simulink model "shift_register_100"  (R2018b)
settings: Solver=FixedStepAuto  StartTime=0.0  StopTime=500*(15e-9)  FixedStep=15e-9  RelTol=1e-3
settings Model: Creator=meyer  LastModifiedBy=jason
settings OptimizationCC: DefaultParameterBehavior=Inlined

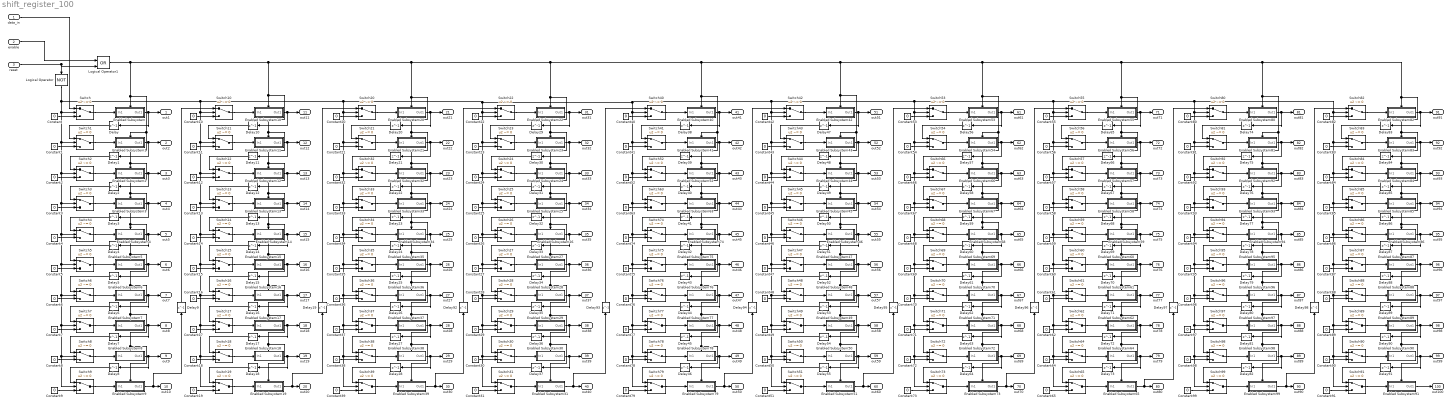
== system shift_register_100 ==
  data_in : Inport  OutDataTypeStr=fixdt(1,16,15)
  enable : Inport  Port=2
  reset : Inport  Port=3
  Constant{,1..99} (100 alike) : Constant  Value=0  OutDataTypeStr=Inherit: Inherit via back propagation  SampleTime=-1
  Delay{,1..98} (99 alike) : Delay  DelayLength=1
  Enabled Subsystem : Subsystem  TreatAsAtomicUnit=on
  Enabled Subsystem1 : Subsystem  TreatAsAtomicUnit=on
  Enabled Subsystem10 : Subsystem  TreatAsAtomicUnit=on
  Enabled Subsystem11 : Subsystem  TreatAsAtomicUnit=on
  Enabled Subsystem12 : Subsystem  TreatAsAtomicUnit=on
  Enabled Subsystem13 : Subsystem  TreatAsAtomicUnit=on
  Enabled Subsystem14 : Subsystem  TreatAsAtomicUnit=on
  Enabled Subsystem15 : Subsystem  TreatAsAtomicUnit=on
  Enabled Subsystem16 : Subsystem  TreatAsAtomicUnit=on
  Enabled Subsystem17 : Subsystem  TreatAsAtomicUnit=on
  Enabled Subsystem18 : Subsystem  TreatAsAtomicUnit=on
  Enabled Subsystem19 : Subsystem  TreatAsAtomicUnit=on
  Enabled Subsystem2 : Subsystem  TreatAsAtomicUnit=on
  Enabled Subsystem20 : Subsystem  TreatAsAtomicUnit=on
  Enabled Subsystem21 : Subsystem  TreatAsAtomicUnit=on
  Enabled Subsystem22 : Subsystem  TreatAsAtomicUnit=on
  Enabled Subsystem23 : Subsystem  TreatAsAtomicUnit=on
  Enabled Subsystem24 : Subsystem  TreatAsAtomicUnit=on
  Enabled Subsystem25 : Subsystem  TreatAsAtomicUnit=on
  Enabled Subsystem26 : Subsystem  TreatAsAtomicUnit=on
  Enabled Subsystem27 : Subsystem  TreatAsAtomicUnit=on
  Enabled Subsystem28 : Subsystem  TreatAsAtomicUnit=on
  Enabled Subsystem29 : Subsystem  TreatAsAtomicUnit=on
  Enabled Subsystem3 : Subsystem  TreatAsAtomicUnit=on
  Enabled Subsystem30 : Subsystem  TreatAsAtomicUnit=on
  Enabled Subsystem31 : Subsystem  TreatAsAtomicUnit=on
  Enabled Subsystem32 : Subsystem  TreatAsAtomicUnit=on
  Enabled Subsystem33 : Subsystem  TreatAsAtomicUnit=on
  Enabled Subsystem34 : Subsystem  TreatAsAtomicUnit=on
  Enabled Subsystem35 : Subsystem  TreatAsAtomicUnit=on
  Enabled Subsystem36 : Subsystem  TreatAsAtomicUnit=on
  Enabled Subsystem37 : Subsystem  TreatAsAtomicUnit=on
  Enabled Subsystem38 : Subsystem  TreatAsAtomicUnit=on
  Enabled Subsystem39 : Subsystem  TreatAsAtomicUnit=on
  Enabled Subsystem4 : Subsystem  TreatAsAtomicUnit=on
  Enabled Subsystem40 : Subsystem  TreatAsAtomicUnit=on
  Enabled Subsystem41 : Subsystem  TreatAsAtomicUnit=on
  Enabled Subsystem42 : Subsystem  TreatAsAtomicUnit=on
  Enabled Subsystem43 : Subsystem  TreatAsAtomicUnit=on
  Enabled Subsystem44 : Subsystem  TreatAsAtomicUnit=on
  Enabled Subsystem45 : Subsystem  TreatAsAtomicUnit=on
  Enabled Subsystem46 : Subsystem  TreatAsAtomicUnit=on
  Enabled Subsystem47 : Subsystem  TreatAsAtomicUnit=on
  Enabled Subsystem48 : Subsystem  TreatAsAtomicUnit=on
  Enabled Subsystem49 : Subsystem  TreatAsAtomicUnit=on
  Enabled Subsystem5 : Subsystem  TreatAsAtomicUnit=on
  Enabled Subsystem50 : Subsystem  TreatAsAtomicUnit=on
  Enabled Subsystem51 : Subsystem  TreatAsAtomicUnit=on
  Enabled Subsystem52 : Subsystem  TreatAsAtomicUnit=on
  Enabled Subsystem53 : Subsystem  TreatAsAtomicUnit=on
  Enabled Subsystem54 : Subsystem  TreatAsAtomicUnit=on
  Enabled Subsystem55 : Subsystem  TreatAsAtomicUnit=on
  Enabled Subsystem56 : Subsystem  TreatAsAtomicUnit=on
  Enabled Subsystem57 : Subsystem  TreatAsAtomicUnit=on
  Enabled Subsystem58 : Subsystem  TreatAsAtomicUnit=on
  Enabled Subsystem59 : Subsystem  TreatAsAtomicUnit=on
  Enabled Subsystem6 : Subsystem  TreatAsAtomicUnit=on
  Enabled Subsystem60 : Subsystem  TreatAsAtomicUnit=on
  Enabled Subsystem61 : Subsystem  TreatAsAtomicUnit=on
  Enabled Subsystem62 : Subsystem  TreatAsAtomicUnit=on
  Enabled Subsystem63 : Subsystem  TreatAsAtomicUnit=on
  Enabled Subsystem64 : Subsystem  TreatAsAtomicUnit=on
  Enabled Subsystem65 : Subsystem  TreatAsAtomicUnit=on
  Enabled Subsystem66 : Subsystem  TreatAsAtomicUnit=on
  Enabled Subsystem67 : Subsystem  TreatAsAtomicUnit=on
  Enabled Subsystem68 : Subsystem  TreatAsAtomicUnit=on
  Enabled Subsystem69 : Subsystem  TreatAsAtomicUnit=on
  Enabled Subsystem7 : Subsystem  TreatAsAtomicUnit=on
  Enabled Subsystem70 : Subsystem  TreatAsAtomicUnit=on
  Enabled Subsystem71 : Subsystem  TreatAsAtomicUnit=on
  Enabled Subsystem72 : Subsystem  TreatAsAtomicUnit=on
  Enabled Subsystem73 : Subsystem  TreatAsAtomicUnit=on
  Enabled Subsystem74 : Subsystem  TreatAsAtomicUnit=on
  Enabled Subsystem75 : Subsystem  TreatAsAtomicUnit=on
  Enabled Subsystem76 : Subsystem  TreatAsAtomicUnit=on
  Enabled Subsystem77 : Subsystem  TreatAsAtomicUnit=on
  Enabled Subsystem78 : Subsystem  TreatAsAtomicUnit=on
  Enabled Subsystem79 : Subsystem  TreatAsAtomicUnit=on
  Enabled Subsystem8 : Subsystem  TreatAsAtomicUnit=on
  Enabled Subsystem80 : Subsystem  TreatAsAtomicUnit=on
  Enabled Subsystem81 : Subsystem  TreatAsAtomicUnit=on
  Enabled Subsystem82 : Subsystem  TreatAsAtomicUnit=on
  Enabled Subsystem83 : Subsystem  TreatAsAtomicUnit=on
  Enabled Subsystem84 : Subsystem  TreatAsAtomicUnit=on
  Enabled Subsystem85 : Subsystem  TreatAsAtomicUnit=on
  Enabled Subsystem86 : Subsystem  TreatAsAtomicUnit=on
  Enabled Subsystem87 : Subsystem  TreatAsAtomicUnit=on
  Enabled Subsystem88 : Subsystem  TreatAsAtomicUnit=on
  Enabled Subsystem89 : Subsystem  TreatAsAtomicUnit=on
  Enabled Subsystem9 : Subsystem  TreatAsAtomicUnit=on
  Enabled Subsystem90 : Subsystem  TreatAsAtomicUnit=on
  Enabled Subsystem91 : Subsystem  TreatAsAtomicUnit=on
  Enabled Subsystem92 : Subsystem  TreatAsAtomicUnit=on
  Enabled Subsystem93 : Subsystem  TreatAsAtomicUnit=on
  Enabled Subsystem94 : Subsystem  TreatAsAtomicUnit=on
  Enabled Subsystem95 : Subsystem  TreatAsAtomicUnit=on
  Enabled Subsystem96 : Subsystem  TreatAsAtomicUnit=on
  Enabled Subsystem97 : Subsystem  TreatAsAtomicUnit=on
  Enabled Subsystem98 : Subsystem  TreatAsAtomicUnit=on
  Enabled Subsystem99 : Subsystem  TreatAsAtomicUnit=on
  Logical Operator : Logic  Operator=NOT  IconShape=distinctive  AllPortsSameDT=off  OutDataTypeStr=boolean
  Logical Operator1 : Logic  Operator=OR  IconShape=distinctive  AllPortsSameDT=off  OutDataTypeStr=boolean
  Switch{,1..99} (100 alike) : Switch  Criteria=u2 ~= 0  OutDataTypeStr=Inherit: Inherit via back propagation
  out1 : Outport
  out2 : Outport  Port=2
  out3 : Outport  Port=3
  out4 : Outport  Port=4
  out5 : Outport  Port=5
  out6 : Outport  Port=6
  out7 : Outport  Port=7
  out8 : Outport  Port=8
  out9 : Outport  Port=9
  out10 : Outport  Port=10
  out11 : Outport  Port=11
  out12 : Outport  Port=12
  out13 : Outport  Port=13
  out14 : Outport  Port=14
  out15 : Outport  Port=15
  out16 : Outport  Port=16
  out17 : Outport  Port=17
  out18 : Outport  Port=18
  out19 : Outport  Port=19
  out20 : Outport  Port=20
  out21 : Outport  Port=21
  out22 : Outport  Port=22
  out23 : Outport  Port=23
  out24 : Outport  Port=24
  out25 : Outport  Port=25
  out26 : Outport  Port=26
  out27 : Outport  Port=27
  out28 : Outport  Port=28
  out29 : Outport  Port=29
  out30 : Outport  Port=30
  out31 : Outport  Port=31
  out32 : Outport  Port=32
  out33 : Outport  Port=33
  out34 : Outport  Port=34
  out35 : Outport  Port=35
  out36 : Outport  Port=36
  out37 : Outport  Port=37
  out38 : Outport  Port=38
  out39 : Outport  Port=39
  out40 : Outport  Port=40
  out41 : Outport  Port=41
  out42 : Outport  Port=42
  out43 : Outport  Port=43
  out44 : Outport  Port=44
  out45 : Outport  Port=45
  out46 : Outport  Port=46
  out47 : Outport  Port=47
  out48 : Outport  Port=48
  out49 : Outport  Port=49
  out50 : Outport  Port=50
  out51 : Outport  Port=51
  out52 : Outport  Port=52
  out53 : Outport  Port=53
  out54 : Outport  Port=54
  out55 : Outport  Port=55
  out56 : Outport  Port=56
  out57 : Outport  Port=57
  out58 : Outport  Port=58
  out59 : Outport  Port=59
  out60 : Outport  Port=60
  out61 : Outport  Port=61
  out62 : Outport  Port=62
  out63 : Outport  Port=63
  out64 : Outport  Port=64
  out65 : Outport  Port=65
  out66 : Outport  Port=66
  out67 : Outport  Port=67
  out68 : Outport  Port=68
  out69 : Outport  Port=69
  out70 : Outport  Port=70
  out71 : Outport  Port=71
  out72 : Outport  Port=72
  out73 : Outport  Port=73
  out74 : Outport  Port=74
  out75 : Outport  Port=75
  out76 : Outport  Port=76
  out77 : Outport  Port=77
  out78 : Outport  Port=78
  out79 : Outport  Port=79
  out80 : Outport  Port=80
  out81 : Outport  Port=81
  out82 : Outport  Port=82
  out83 : Outport  Port=83
  out84 : Outport  Port=84
  out85 : Outport  Port=85
  out86 : Outport  Port=86
  out87 : Outport  Port=87
  out88 : Outport  Port=88
  out89 : Outport  Port=89
  out90 : Outport  Port=90
  out91 : Outport  Port=91
  out92 : Outport  Port=92
  out93 : Outport  Port=93
  out94 : Outport  Port=94
  out95 : Outport  Port=95
  out96 : Outport  Port=96
  out97 : Outport  Port=97
  out98 : Outport  Port=98
  out99 : Outport  Port=99
  out100 : Outport  Port=100
  wires:
  Constant/1 -> Switch/3
  reset/1 -> Logical Operator1/2, Logical Operator/1
  data_in/1 -> Switch/1
  Switch/1 -> Enabled Subsystem/1(In1)
  Constant1/1 -> Switch1/3
  Switch1/1 -> Enabled Subsystem1/1(In1)
  Switch2/1 -> Enabled Subsystem2/1(In1)
  Constant2/1 -> Switch2/3
  Enabled Subsystem1/1(Out1) -> Delay1/1, out2/1
  Switch3/1 -> Enabled Subsystem3/1(In1)
  Enabled Subsystem2/1(Out1) -> Delay2/1, out3/1
  Constant3/1 -> Switch3/3
  Enabled Subsystem3/1(Out1) -> Delay3/1, out4/1
  Switch4/1 -> Enabled Subsystem4/1(In1)
  Constant4/1 -> Switch4/3
  Enabled Subsystem/1(Out1) -> Delay/1, out1/1
  Switch5/1 -> Enabled Subsystem5/1(In1)
  Constant5/1 -> Switch5/3
  Enabled Subsystem4/1(Out1) -> Delay4/1, out5/1
  Constant6/1 -> Switch6/3
  Enabled Subsystem5/1(Out1) -> Delay5/1, out6/1
  Switch6/1 -> Enabled Subsystem6/1(In1)
  Switch7/1 -> Enabled Subsystem7/1(In1)
  Enabled Subsystem6/1(Out1) -> Delay6/1, out7/1
  Constant7/1 -> Switch7/3
  Enabled Subsystem7/1(Out1) -> Delay7/1, out8/1
  Switch8/1 -> Enabled Subsystem8/1(In1)
  Constant8/1 -> Switch8/3
  Enabled Subsystem8/1(Out1) -> Delay8/1, out9/1
  Switch9/1 -> Enabled Subsystem9/1(In1)
  Constant9/1 -> Switch9/3
  Enabled Subsystem16/1(Out1) -> Delay16/1, out17/1
  Switch14/1 -> Enabled Subsystem14/1(In1)
  Enabled Subsystem15/1(Out1) -> Delay15/1, out16/1
  Enabled Subsystem12/1(Out1) -> Delay12/1, out13/1
  Switch12/1 -> Enabled Subsystem12/1(In1)
  Constant12/1 -> Switch12/3
  Switch17/1 -> Enabled Subsystem17/1(In1)
  Constant17/1 -> Switch17/3
  Enabled Subsystem9/1(Out1) -> Delay9/1, out10/1
  Switch10/1 -> Enabled Subsystem10/1(In1)
  Enabled Subsystem13/1(Out1) -> Delay13/1, out14/1
  Switch11/1 -> Enabled Subsystem11/1(In1)
  Switch13/1 -> Enabled Subsystem13/1(In1)
  Constant13/1 -> Switch13/3
  Switch18/1 -> Enabled Subsystem18/1(In1)
  Constant18/1 -> Switch18/3
  Constant15/1 -> Switch15/3
  Enabled Subsystem11/1(Out1) -> Delay11/1, out12/1
  Constant10/1 -> Switch10/3
  Enabled Subsystem18/1(Out1) -> Delay18/1, out19/1
  Constant19/1 -> Switch19/3
  Constant14/1 -> Switch14/3
  Enabled Subsystem17/1(Out1) -> Delay17/1, out18/1
  Switch16/1 -> Enabled Subsystem16/1(In1)
  Enabled Subsystem10/1(Out1) -> Delay10/1, out11/1
  Constant16/1 -> Switch16/3
  Constant11/1 -> Switch11/3
  Switch19/1 -> Enabled Subsystem19/1(In1)
  Enabled Subsystem14/1(Out1) -> Delay14/1, out15/1
  Switch15/1 -> Enabled Subsystem15/1(In1)
  Enabled Subsystem36/1(Out1) -> Delay26/1, out27/1
  Constant34/1 -> Switch34/3
  Switch34/1 -> Enabled Subsystem34/1(In1)
  Enabled Subsystem35/1(Out1) -> Delay25/1, out26/1
  Enabled Subsystem33/1(Out1) -> Delay23/1, out24/1
  Switch35/1 -> Enabled Subsystem35/1(In1)
  Enabled Subsystem32/1(Out1) -> Delay22/1, out23/1
  Switch32/1 -> Enabled Subsystem32/1(In1)
  Constant32/1 -> Switch32/3
  Constant39/1 -> Switch39/3
  Switch37/1 -> Enabled Subsystem37/1(In1)
  Switch39/1 -> Enabled Subsystem39/1(In1)
  Enabled Subsystem19/1(Out1) -> Delay19/1, out20/1
  Switch20/1 -> Enabled Subsystem20/1(In1)
  Constant28/1 -> Switch28/3
  Constant23/1 -> Switch23/3
  Enabled Subsystem22/1(Out1) -> Delay29/1, out31/1
  Switch28/1 -> Enabled Subsystem28/1(In1)
  Enabled Subsystem29/1(Out1) -> Delay36/1, out38/1
  Constant26/1 -> Switch26/3
  Constant35/1 -> Switch35/3
  Constant37/1 -> Switch37/3
  Constant31/1 -> Switch31/3
  Enabled Subsystem30/1(Out1) -> Delay37/1, out39/1
  Switch33/1 -> Enabled Subsystem33/1(In1)
  Constant27/1 -> Switch27/3
  Constant30/1 -> Switch30/3
  Constant25/1 -> Switch25/3
  Constant38/1 -> Switch38/3
  Enabled Subsystem26/1(Out1) -> Delay33/1, out35/1
  Switch21/1 -> Enabled Subsystem21/1(In1)
  Switch38/1 -> Enabled Subsystem38/1(In1)
  Constant22/1 -> Switch22/3
  Switch31/1 -> Enabled Subsystem31/1(In1)
  Switch22/1 -> Enabled Subsystem22/1(In1)
  Enabled Subsystem25/1(Out1) -> Delay32/1, out34/1
  Switch26/1 -> Enabled Subsystem26/1(In1)
  Constant20/1 -> Switch20/3
  Enabled Subsystem20/1(Out1) -> Delay20/1, out21/1
  Enabled Subsystem37/1(Out1) -> Delay27/1, out28/1
  Switch27/1 -> Enabled Subsystem27/1(In1)
  Switch30/1 -> Enabled Subsystem30/1(In1)
  Enabled Subsystem38/1(Out1) -> Delay28/1, out29/1
  Enabled Subsystem27/1(Out1) -> Delay34/1, out36/1
  Constant33/1 -> Switch33/3
  Constant29/1 -> Switch29/3
  Switch25/1 -> Enabled Subsystem25/1(In1)
  Switch23/1 -> Enabled Subsystem23/1(In1)
  Switch29/1 -> Enabled Subsystem29/1(In1)
  Constant24/1 -> Switch24/3
  Enabled Subsystem39/1(Out1) -> Delay92/1, out30/1
  Switch24/1 -> Enabled Subsystem24/1(In1)
  Switch36/1 -> Enabled Subsystem36/1(In1)
  Constant36/1 -> Switch36/3
  Enabled Subsystem24/1(Out1) -> Delay31/1, out33/1
  Constant21/1 -> Switch21/3
  Enabled Subsystem23/1(Out1) -> Delay30/1, out32/1
  Enabled Subsystem21/1(Out1) -> Delay21/1, out22/1
  Enabled Subsystem28/1(Out1) -> Delay35/1, out37/1
  Enabled Subsystem34/1(Out1) -> Delay24/1, out25/1
  enable/1 -> Logical Operator1/1
  Enabled Subsystem76/1(Out1) -> Delay44/1, out47/1
  Enabled Subsystem54/1(Out1) -> Delay57/1, out62/1
  Switch57/1 -> Enabled Subsystem57/1(In1)
  Switch70/1 -> Enabled Subsystem70/1(In1)
  Constant57/1 -> Switch57/3
  Switch56/1 -> Enabled Subsystem56/1(In1)
  Constant67/1 -> Switch67/3
  Enabled Subsystem60/1(Out1) -> Delay70/1, out76/1
  Switch58/1 -> Enabled Subsystem58/1(In1)
  Enabled Subsystem72/1(Out1) -> Delay64/1, out69/1
  Enabled Subsystem71/1(Out1) -> Delay63/1, out68/1
  Constant54/1 -> Switch54/3
  Enabled Subsystem57/1(Out1) -> Delay67/1, out73/1
  Enabled Subsystem68/1(Out1) -> Delay60/1, out65/1
  Enabled Subsystem61/1(Out1) -> Delay71/1, out77/1
  Constant74/1 -> Switch74/3
  Switch74/1 -> Enabled Subsystem74/1(In1)
  Switch55/1 -> Enabled Subsystem55/1(In1)
  Switch59/1 -> Enabled Subsystem59/1(In1)
  Constant55/1 -> Switch55/3
  Enabled Subsystem58/1(Out1) -> Delay68/1, out74/1
  Constant58/1 -> Switch58/3
  Constant53/1 -> Switch53/3
  Enabled Subsystem59/1(Out1) -> Delay69/1, out75/1
  Constant72/1 -> Switch72/3
  Switch54/1 -> Enabled Subsystem54/1(In1)
  Constant69/1 -> Switch69/3
  Switch67/1 -> Enabled Subsystem67/1(In1)
  Constant64/1 -> Switch64/3
  Constant71/1 -> Switch71/3
  Switch64/1 -> Enabled Subsystem64/1(In1)
  Constant65/1 -> Switch65/3
  Switch65/1 -> Enabled Subsystem65/1(In1)
  Switch61/1 -> Enabled Subsystem61/1(In1)
  Constant61/1 -> Switch61/3
  Constant56/1 -> Switch56/3
  Switch53/1 -> Enabled Subsystem53/1(In1)
  Switch73/1 -> Enabled Subsystem73/1(In1)
  Switch66/1 -> Enabled Subsystem66/1(In1)
  Constant73/1 -> Switch73/3
  Switch71/1 -> Enabled Subsystem71/1(In1)
  Switch69/1 -> Enabled Subsystem69/1(In1)
  Enabled Subsystem67/1(Out1) -> Delay59/1, out64/1
  Enabled Subsystem62/1(Out1) -> Delay72/1, out78/1
  Enabled Subsystem70/1(Out1) -> Delay62/1, out67/1
  Enabled Subsystem75/1(Out1) -> Delay43/1, out46/1
  Enabled Subsystem53/1(Out1) -> Delay56/1, out61/1
  Enabled Subsystem63/1(Out1) -> Delay41/1, out44/1
  Switch75/1 -> Enabled Subsystem75/1(In1)
  Constant66/1 -> Switch66/3
  Constant59/1 -> Switch59/3
  Enabled Subsystem52/1(Out1) -> Delay40/1, out43/1
  Switch52/1 -> Enabled Subsystem52/1(In1)
  Constant52/1 -> Switch52/3
  Constant79/1 -> Switch79/3
  Switch77/1 -> Enabled Subsystem77/1(In1)
  Switch79/1 -> Enabled Subsystem79/1(In1)
  Enabled Subsystem31/1(Out1) -> Delay93/1, out40/1
  Switch40/1 -> Enabled Subsystem40/1(In1)
  Constant48/1 -> Switch48/3
  Constant43/1 -> Switch43/3
  Enabled Subsystem42/1(Out1) -> Delay47/1, out51/1
  Enabled Subsystem73/1(Out1) -> Delay96/1, out70/1
  Constant62/1 -> Switch62/3
  Switch48/1 -> Enabled Subsystem48/1(In1)
  Enabled Subsystem49/1(Out1) -> Delay54/1, out58/1
  Enabled Subsystem56/1(Out1) -> Delay66/1, out72/1
  Constant46/1 -> Switch46/3
  Constant75/1 -> Switch75/3
  Constant77/1 -> Switch77/3
  Enabled Subsystem55/1(Out1) -> Delay65/1, out71/1
  Switch68/1 -> Enabled Subsystem68/1(In1)
  Enabled Subsystem69/1(Out1) -> Delay61/1, out66/1
  Switch72/1 -> Enabled Subsystem72/1(In1)
  Constant70/1 -> Switch70/3
  Constant51/1 -> Switch51/3
  Enabled Subsystem50/1(Out1) -> Delay55/1, out59/1
  Constant63/1 -> Switch63/3
  Constant42/1 -> Switch42/3
  Enabled Subsystem51/1(Out1) -> Delay95/1, out60/1
  Enabled Subsystem43/1(Out1) -> Delay48/1, out52/1
  Constant47/1 -> Switch47/3
  Constant50/1 -> Switch50/3
  Switch43/1 -> Enabled Subsystem43/1(In1)
  Switch78/1 -> Enabled Subsystem78/1(In1)
  Switch45/1 -> Enabled Subsystem45/1(In1)
  Constant45/1 -> Switch45/3
  Enabled Subsystem46/1(Out1) -> Delay51/1, out55/1
  Switch41/1 -> Enabled Subsystem41/1(In1)
  Switch42/1 -> Enabled Subsystem42/1(In1)
  Switch46/1 -> Enabled Subsystem46/1(In1)
  Enabled Subsystem45/1(Out1) -> Delay50/1, out54/1
  Switch60/1 -> Enabled Subsystem60/1(In1)
  Enabled Subsystem40/1(Out1) -> Delay38/1, out41/1
  Constant60/1 -> Switch60/3
  Enabled Subsystem77/1(Out1) -> Delay45/1, out48/1
  Switch47/1 -> Enabled Subsystem47/1(In1)
  Enabled Subsystem66/1(Out1) -> Delay58/1, out63/1
  Switch62/1 -> Enabled Subsystem62/1(In1)
  Enabled Subsystem78/1(Out1) -> Delay46/1, out49/1
  Switch50/1 -> Enabled Subsystem50/1(In1)
  Switch49/1 -> Enabled Subsystem49/1(In1)
  Constant44/1 -> Switch44/3
  Enabled Subsystem79/1(Out1) -> Delay94/1, out50/1
  Switch44/1 -> Enabled Subsystem44/1(In1)
  Enabled Subsystem64/1(Out1) -> Delay73/1, out79/1
  Enabled Subsystem47/1(Out1) -> Delay52/1, out56/1
  Switch63/1 -> Enabled Subsystem63/1(In1)
  Switch51/1 -> Enabled Subsystem51/1(In1)
  Constant78/1 -> Switch78/3
  Switch76/1 -> Enabled Subsystem76/1(In1)
  Constant76/1 -> Switch76/3
  Constant40/1 -> Switch40/3
  Enabled Subsystem44/1(Out1) -> Delay49/1, out53/1
  Constant41/1 -> Switch41/3
  Enabled Subsystem41/1(Out1) -> Delay39/1, out42/1
  Enabled Subsystem48/1(Out1) -> Delay53/1, out57/1
  Constant68/1 -> Switch68/3
  Enabled Subsystem74/1(Out1) -> Delay42/1, out45/1
  Constant49/1 -> Switch49/3
  Constant94/1 -> Switch94/3
  Switch89/1 -> Enabled Subsystem89/1(In1)
  Constant87/1 -> Switch87/3
  Switch87/1 -> Enabled Subsystem87/1(In1)
  Enabled Subsystem91/1(Out1) -> out100/1
  Enabled Subsystem65/1(Out1) -> Delay97/1, out80/1
  Constant96/1 -> Switch96/3
  Switch94/1 -> Enabled Subsystem94/1(In1)
  Switch98/1 -> Enabled Subsystem98/1(In1)
  Enabled Subsystem95/1(Out1) -> Delay79/1, out86/1
  Enabled Subsystem83/1(Out1) -> Delay84/1, out92/1
  Enabled Subsystem99/1(Out1) -> Delay98/1, out90/1
  Logical Operator/1 -> Switch91/2, Switch90/2, Switch89/2, Switch88/2, Switch87/2, Switch86/2, Switch85/2, Switch84/2, Switch83/2, Switch82/2, Switch99/2, Switch98/2, Switch97/2, Switch96/2, Switch95/2, Switch94/2, Switch93/2, Switch92/2, Switch81/2, Switch80/2, Switch65/2, Switch64/2, Switch62/2, Switch61/2, Switch60/2, Switch59/2, Switch58/2, Switch57/2, Switch56/2, Switch55/2, Switch73/2, Switch72/2, Switch71/2, Switch70/2, Switch69/2, Switch68/2, Switch67/2, Switch66/2, Switch54/2, Switch53/2, Switch51/2, Switch50/2, Switch49/2, Switch48/2, Switch47/2, Switch46/2, Switch45/2, Switch44/2, Switch43/2, Switch42/2, Switch79/2, Switch78/2, Switch77/2, Switch76/2, Switch75/2, Switch74/2, Switch63/2, Switch52/2, Switch41/2, Switch40/2, Switch31/2, Switch30/2, Switch29/2, Switch28/2, Switch27/2, Switch26/2, Switch25/2, Switch24/2, Switch23/2, Switch22/2, Switch39/2, Switch38/2, Switch37/2, Switch36/2, Switch35/2, Switch34/2, Switch33/2, Switch32/2, Switch21/2, Switch20/2, Switch19/2, Switch18/2, Switch17/2, Switch16/2, Switch15/2, Switch14/2, Switch13/2, Switch12/2, Switch11/2, Switch10/2, Switch9/2, Switch8/2, Switch7/2, Switch6/2, Switch5/2, Switch4/2, Switch3/2, Switch2/2, Switch1/2, Switch/2
  Constant92/1 -> Switch92/3
  Enabled Subsystem80/1(Out1) -> Delay74/1, out81/1
  Enabled Subsystem90/1(Out1) -> Delay91/1, out99/1
  Enabled Subsystem92/1(Out1) -> Delay76/1, out83/1
  Enabled Subsystem93/1(Out1) -> Delay77/1, out84/1
  Enabled Subsystem96/1(Out1) -> Delay80/1, out87/1
  Enabled Subsystem89/1(Out1) -> Delay90/1, out98/1
  Constant99/1 -> Switch99/3
  Switch97/1 -> Enabled Subsystem97/1(In1)
  Constant88/1 -> Switch88/3
  Constant83/1 -> Switch83/3
  Switch90/1 -> Enabled Subsystem90/1(In1)
  Switch91/1 -> Enabled Subsystem91/1(In1)
  Switch99/1 -> Enabled Subsystem99/1(In1)
  Enabled Subsystem85/1(Out1) -> Delay86/1, out94/1
  Constant80/1 -> Switch80/3
  Enabled Subsystem86/1(Out1) -> Delay87/1, out95/1
  Constant85/1 -> Switch85/3
  Switch92/1 -> Enabled Subsystem92/1(In1)
  Enabled Subsystem84/1(Out1) -> Delay85/1, out93/1
  Constant90/1 -> Switch90/3
  Enabled Subsystem94/1(Out1) -> Delay78/1, out85/1
  Switch88/1 -> Enabled Subsystem88/1(In1)
  Enabled Subsystem88/1(Out1) -> Delay89/1, out97/1
  Switch81/1 -> Enabled Subsystem81/1(In1)
  Constant98/1 -> Switch98/3
  Constant86/1 -> Switch86/3
  Switch85/1 -> Enabled Subsystem85/1(In1)
  Constant89/1 -> Switch89/3
  Constant91/1 -> Switch91/3
  Constant84/1 -> Switch84/3
  Constant93/1 -> Switch93/3
  Switch96/1 -> Enabled Subsystem96/1(In1)
  Switch95/1 -> Enabled Subsystem95/1(In1)
  Switch83/1 -> Enabled Subsystem83/1(In1)
  Switch80/1 -> Enabled Subsystem80/1(In1)
  Switch84/1 -> Enabled Subsystem84/1(In1)
  Enabled Subsystem87/1(Out1) -> Delay88/1, out96/1
  Constant81/1 -> Switch81/3
  Constant95/1 -> Switch95/3
  Enabled Subsystem98/1(Out1) -> Delay82/1, out89/1
  Enabled Subsystem81/1(Out1) -> Delay75/1, out82/1
  Logical Operator1/1 -> Enabled Subsystem/Enable, Enabled Subsystem1/Enable, Enabled Subsystem9/Enable, Enabled Subsystem8/Enable, Enabled Subsystem7/Enable, Enabled Subsystem6/Enable, Enabled Subsystem5/Enable, Enabled Subsystem4/Enable, Enabled Subsystem3/Enable, Enabled Subsystem2/Enable, Enabled Subsystem81/Enable, Enabled Subsystem99/Enable, Enabled Subsystem98/Enable, Enabled Subsystem97/Enable, Enabled Subsystem96/Enable, Enabled Subsystem95/Enable, Enabled Subsystem94/Enable, Enabled Subsystem93/Enable, Enabled Subsystem92/Enable, Enabled Subsystem80/Enable, Enabled Subsystem91/Enable, Enabled Subsystem90/Enable, Enabled Subsystem89/Enable, Enabled Subsystem88/Enable, Enabled Subsystem87/Enable, Enabled Subsystem86/Enable, Enabled Subsystem85/Enable, Enabled Subsystem84/Enable, Enabled Subsystem83/Enable, Enabled Subsystem82/Enable, Enabled Subsystem65/Enable, Enabled Subsystem64/Enable, Enabled Subsystem62/Enable, Enabled Subsystem61/Enable, Enabled Subsystem60/Enable, Enabled Subsystem59/Enable, Enabled Subsystem58/Enable, Enabled Subsystem57/Enable, Enabled Subsystem56/Enable, Enabled Subsystem55/Enable, Enabled Subsystem54/Enable, Enabled Subsystem73/Enable, Enabled Subsystem72/Enable, Enabled Subsystem71/Enable, Enabled Subsystem70/Enable, Enabled Subsystem69/Enable, Enabled Subsystem68/Enable, Enabled Subsystem67/Enable, Enabled Subsystem66/Enable, Enabled Subsystem53/Enable, Enabled Subsystem43/Enable, Enabled Subsystem51/Enable, Enabled Subsystem50/Enable, Enabled Subsystem49/Enable, Enabled Subsystem48/Enable, Enabled Subsystem47/Enable, Enabled Subsystem46/Enable, Enabled Subsystem45/Enable, Enabled Subsystem44/Enable, Enabled Subsystem42/Enable, Enabled Subsystem41/Enable, Enabled Subsystem79/Enable, Enabled Subsystem78/Enable, Enabled Subsystem77/Enable, Enabled Subsystem76/Enable, Enabled Subsystem75/Enable, Enabled Subsystem74/Enable, Enabled Subsystem63/Enable, Enabled Subsystem52/Enable, Enabled Subsystem40/Enable, Enabled Subsystem31/Enable, Enabled Subsystem30/Enable, Enabled Subsystem29/Enable, Enabled Subsystem28/Enable, Enabled Subsystem27/Enable, Enabled Subsystem26/Enable, Enabled Subsystem25/Enable, Enabled Subsystem24/Enable, Enabled Subsystem23/Enable, Enabled Subsystem22/Enable, Enabled Subsystem39/Enable, Enabled Subsystem38/Enable, Enabled Subsystem37/Enable, Enabled Subsystem36/Enable, Enabled Subsystem35/Enable, Enabled Subsystem34/Enable, Enabled Subsystem33/Enable, Enabled Subsystem32/Enable, Enabled Subsystem21/Enable, Enabled Subsystem20/Enable, Enabled Subsystem10/Enable, Enabled Subsystem19/Enable, Enabled Subsystem18/Enable, Enabled Subsystem17/Enable, Enabled Subsystem16/Enable, Enabled Subsystem15/Enable, Enabled Subsystem14/Enable, Enabled Subsystem13/Enable, Enabled Subsystem12/Enable, Enabled Subsystem11/Enable
  Enabled Subsystem82/1(Out1) -> Delay83/1, out91/1
  Constant97/1 -> Switch97/3
  Enabled Subsystem97/1(Out1) -> Delay81/1, out88/1
  Constant82/1 -> Switch82/3
  Switch93/1 -> Enabled Subsystem93/1(In1)
  Switch86/1 -> Enabled Subsystem86/1(In1)
  Switch82/1 -> Enabled Subsystem82/1(In1)
  Delay/1 -> Switch1/1
  Delay1/1 -> Switch2/1
  Delay2/1 -> Switch3/1
  Delay3/1 -> Switch4/1
  Delay4/1 -> Switch5/1
  Delay5/1 -> Switch6/1
  Delay6/1 -> Switch7/1
  Delay7/1 -> Switch8/1
  Delay8/1 -> Switch9/1
  Delay9/1 -> Switch10/1
  Delay10/1 -> Switch11/1
  Delay11/1 -> Switch12/1
  Delay12/1 -> Switch13/1
  Delay13/1 -> Switch14/1
  Delay14/1 -> Switch15/1
  Delay15/1 -> Switch16/1
  Delay16/1 -> Switch17/1
  Delay17/1 -> Switch18/1
  Delay18/1 -> Switch19/1
  Delay19/1 -> Switch20/1
  Delay20/1 -> Switch21/1
  Delay21/1 -> Switch32/1
  Delay22/1 -> Switch33/1
  Delay23/1 -> Switch34/1
  Delay26/1 -> Switch37/1
  Delay24/1 -> Switch35/1
  Delay25/1 -> Switch36/1
  Delay27/1 -> Switch38/1
  Delay28/1 -> Switch39/1
  Delay30/1 -> Switch24/1
  Delay29/1 -> Switch23/1
  Delay33/1 -> Switch27/1
  Delay35/1 -> Switch29/1
  Delay34/1 -> Switch28/1
  Delay32/1 -> Switch26/1
  Delay31/1 -> Switch25/1
  Delay36/1 -> Switch30/1
  Delay37/1 -> Switch31/1
  Delay38/1 -> Switch41/1
  Delay39/1 -> Switch52/1
  Delay40/1 -> Switch63/1
  Delay42/1 -> Switch75/1
  Delay41/1 -> Switch74/1
  Delay45/1 -> Switch78/1
  Delay46/1 -> Switch79/1
  Delay44/1 -> Switch77/1
  Delay43/1 -> Switch76/1
  Delay48/1 -> Switch44/1
  Delay47/1 -> Switch43/1
  Delay52/1 -> Switch48/1
  Delay49/1 -> Switch45/1
  Delay50/1 -> Switch46/1
  Delay51/1 -> Switch47/1
  Delay55/1 -> Switch51/1
  Delay54/1 -> Switch50/1
  Delay53/1 -> Switch49/1
  Delay58/1 -> Switch67/1
  Delay59/1 -> Switch68/1
  Delay60/1 -> Switch69/1
  Delay61/1 -> Switch70/1
  Delay62/1 -> Switch71/1
  Delay63/1 -> Switch72/1
  Delay64/1 -> Switch73/1
  Delay56/1 -> Switch54/1
  Delay57/1 -> Switch66/1
  Delay65/1 -> Switch56/1
  Delay66/1 -> Switch57/1
  Delay67/1 -> Switch58/1
  Delay68/1 -> Switch59/1
  Delay69/1 -> Switch60/1
  Delay70/1 -> Switch61/1
  Delay71/1 -> Switch62/1
  Delay73/1 -> Switch65/1
  Delay72/1 -> Switch64/1
  Delay75/1 -> Switch92/1
  Delay74/1 -> Switch81/1
  Delay76/1 -> Switch93/1
  Delay77/1 -> Switch94/1
  Delay78/1 -> Switch95/1
  Delay80/1 -> Switch97/1
  Delay79/1 -> Switch96/1
  Delay81/1 -> Switch98/1
  Delay82/1 -> Switch99/1
  Delay83/1 -> Switch83/1
  Delay84/1 -> Switch84/1
  Delay87/1 -> Switch87/1
  Delay86/1 -> Switch86/1
  Delay85/1 -> Switch85/1
  Delay88/1 -> Switch88/1
  Delay89/1 -> Switch89/1
  Delay90/1 -> Switch90/1
  Delay91/1 -> Switch91/1
  Delay92/1 -> Switch22/1
  Delay93/1 -> Switch40/1
  Delay94/1 -> Switch42/1
  Delay95/1 -> Switch53/1
  Delay96/1 -> Switch55/1
  Delay97/1 -> Switch80/1
  Delay98/1 -> Switch82/1

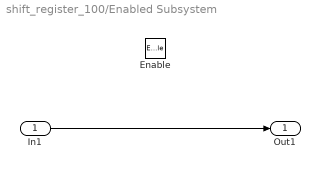
== system shift_register_100/Enabled Subsystem ==
  In1 : Inport
  Enable : EnablePort
  Out1 : Outport  InitialOutput=0
  wires:
  In1/1 -> Out1/1

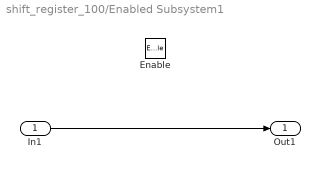
== system shift_register_100/Enabled Subsystem1 ==
  In1 : Inport
  Enable : EnablePort
  Out1 : Outport  InitialOutput=0
  wires:
  In1/1 -> Out1/1

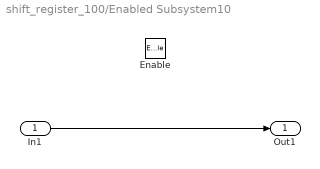
== system shift_register_100/Enabled Subsystem10 ==
  In1 : Inport
  Enable : EnablePort
  Out1 : Outport  InitialOutput=0
  wires:
  In1/1 -> Out1/1

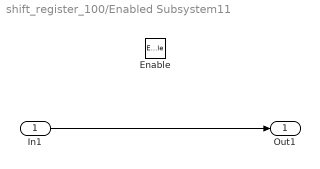
== system shift_register_100/Enabled Subsystem11 ==
  In1 : Inport
  Enable : EnablePort
  Out1 : Outport  InitialOutput=0
  wires:
  In1/1 -> Out1/1

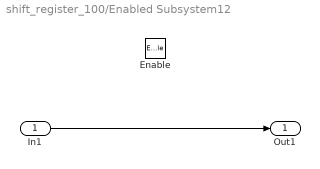
== system shift_register_100/Enabled Subsystem12 ==
  In1 : Inport
  Enable : EnablePort
  Out1 : Outport  InitialOutput=0
  wires:
  In1/1 -> Out1/1

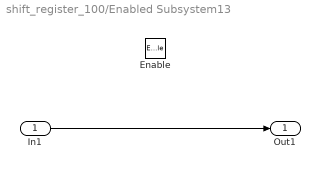
== system shift_register_100/Enabled Subsystem13 ==
  In1 : Inport
  Enable : EnablePort
  Out1 : Outport  InitialOutput=0
  wires:
  In1/1 -> Out1/1

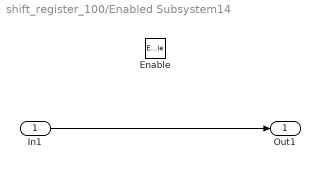
== system shift_register_100/Enabled Subsystem14 ==
  In1 : Inport
  Enable : EnablePort
  Out1 : Outport  InitialOutput=0
  wires:
  In1/1 -> Out1/1

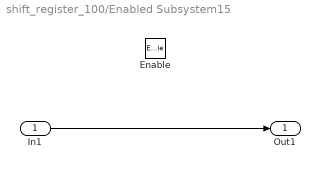
== system shift_register_100/Enabled Subsystem15 ==
  In1 : Inport
  Enable : EnablePort
  Out1 : Outport  InitialOutput=0
  wires:
  In1/1 -> Out1/1

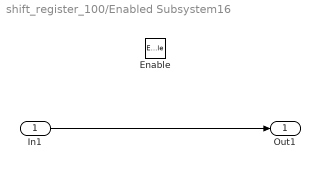
== system shift_register_100/Enabled Subsystem16 ==
  In1 : Inport
  Enable : EnablePort
  Out1 : Outport  InitialOutput=0
  wires:
  In1/1 -> Out1/1

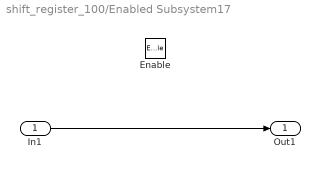
== system shift_register_100/Enabled Subsystem17 ==
  In1 : Inport
  Enable : EnablePort
  Out1 : Outport  InitialOutput=0
  wires:
  In1/1 -> Out1/1

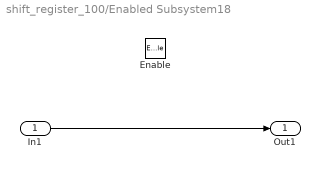
== system shift_register_100/Enabled Subsystem18 ==
  In1 : Inport
  Enable : EnablePort
  Out1 : Outport  InitialOutput=0
  wires:
  In1/1 -> Out1/1

== system shift_register_100/Enabled Subsystem19 ==
  In1 : Inport
  Enable : EnablePort
  Out1 : Outport  InitialOutput=0
  wires:
  In1/1 -> Out1/1

== system shift_register_100/Enabled Subsystem2 ==
  In1 : Inport
  Enable : EnablePort
  Out1 : Outport  InitialOutput=0
  wires:
  In1/1 -> Out1/1

== system shift_register_100/Enabled Subsystem20 ==
  In1 : Inport
  Enable : EnablePort
  Out1 : Outport  InitialOutput=0
  wires:
  In1/1 -> Out1/1

== system shift_register_100/Enabled Subsystem21 ==
  In1 : Inport
  Enable : EnablePort
  Out1 : Outport  InitialOutput=0
  wires:
  In1/1 -> Out1/1

== system shift_register_100/Enabled Subsystem22 ==
  In1 : Inport
  Enable : EnablePort
  Out1 : Outport  InitialOutput=0
  wires:
  In1/1 -> Out1/1

== system shift_register_100/Enabled Subsystem23 ==
  In1 : Inport
  Enable : EnablePort
  Out1 : Outport  InitialOutput=0
  wires:
  In1/1 -> Out1/1

== system shift_register_100/Enabled Subsystem24 ==
  In1 : Inport
  Enable : EnablePort
  Out1 : Outport  InitialOutput=0
  wires:
  In1/1 -> Out1/1

== system shift_register_100/Enabled Subsystem25 ==
  In1 : Inport
  Enable : EnablePort
  Out1 : Outport  InitialOutput=0
  wires:
  In1/1 -> Out1/1

== system shift_register_100/Enabled Subsystem26 ==
  In1 : Inport
  Enable : EnablePort
  Out1 : Outport  InitialOutput=0
  wires:
  In1/1 -> Out1/1

== system shift_register_100/Enabled Subsystem27 ==
  In1 : Inport
  Enable : EnablePort
  Out1 : Outport  InitialOutput=0
  wires:
  In1/1 -> Out1/1

== system shift_register_100/Enabled Subsystem28 ==
  In1 : Inport
  Enable : EnablePort
  Out1 : Outport  InitialOutput=0
  wires:
  In1/1 -> Out1/1

== system shift_register_100/Enabled Subsystem29 ==
  In1 : Inport
  Enable : EnablePort
  Out1 : Outport  InitialOutput=0
  wires:
  In1/1 -> Out1/1

== system shift_register_100/Enabled Subsystem3 ==
  In1 : Inport
  Enable : EnablePort
  Out1 : Outport  InitialOutput=0
  wires:
  In1/1 -> Out1/1

== system shift_register_100/Enabled Subsystem30 ==
  In1 : Inport
  Enable : EnablePort
  Out1 : Outport  InitialOutput=0
  wires:
  In1/1 -> Out1/1

== system shift_register_100/Enabled Subsystem31 ==
  In1 : Inport
  Enable : EnablePort
  Out1 : Outport  InitialOutput=0
  wires:
  In1/1 -> Out1/1

== system shift_register_100/Enabled Subsystem32 ==
  In1 : Inport
  Enable : EnablePort
  Out1 : Outport  InitialOutput=0
  wires:
  In1/1 -> Out1/1

== system shift_register_100/Enabled Subsystem33 ==
  In1 : Inport
  Enable : EnablePort
  Out1 : Outport  InitialOutput=0
  wires:
  In1/1 -> Out1/1

== system shift_register_100/Enabled Subsystem34 ==
  In1 : Inport
  Enable : EnablePort
  Out1 : Outport  InitialOutput=0
  wires:
  In1/1 -> Out1/1

== system shift_register_100/Enabled Subsystem35 ==
  In1 : Inport
  Enable : EnablePort
  Out1 : Outport  InitialOutput=0
  wires:
  In1/1 -> Out1/1

== system shift_register_100/Enabled Subsystem36 ==
  In1 : Inport
  Enable : EnablePort
  Out1 : Outport  InitialOutput=0
  wires:
  In1/1 -> Out1/1

== system shift_register_100/Enabled Subsystem37 ==
  In1 : Inport
  Enable : EnablePort
  Out1 : Outport  InitialOutput=0
  wires:
  In1/1 -> Out1/1

== system shift_register_100/Enabled Subsystem38 ==
  In1 : Inport
  Enable : EnablePort
  Out1 : Outport  InitialOutput=0
  wires:
  In1/1 -> Out1/1

== system shift_register_100/Enabled Subsystem39 ==
  In1 : Inport
  Enable : EnablePort
  Out1 : Outport  InitialOutput=0
  wires:
  In1/1 -> Out1/1

== system shift_register_100/Enabled Subsystem4 ==
  In1 : Inport
  Enable : EnablePort
  Out1 : Outport  InitialOutput=0
  wires:
  In1/1 -> Out1/1

== system shift_register_100/Enabled Subsystem40 ==
  In1 : Inport
  Enable : EnablePort
  Out1 : Outport  InitialOutput=0
  wires:
  In1/1 -> Out1/1

== system shift_register_100/Enabled Subsystem41 ==
  In1 : Inport
  Enable : EnablePort
  Out1 : Outport  InitialOutput=0
  wires:
  In1/1 -> Out1/1

== system shift_register_100/Enabled Subsystem42 ==
  In1 : Inport
  Enable : EnablePort
  Out1 : Outport  InitialOutput=0
  wires:
  In1/1 -> Out1/1

== system shift_register_100/Enabled Subsystem43 ==
  In1 : Inport
  Enable : EnablePort
  Out1 : Outport  InitialOutput=0
  wires:
  In1/1 -> Out1/1

== system shift_register_100/Enabled Subsystem44 ==
  In1 : Inport
  Enable : EnablePort
  Out1 : Outport  InitialOutput=0
  wires:
  In1/1 -> Out1/1

== system shift_register_100/Enabled Subsystem45 ==
  In1 : Inport
  Enable : EnablePort
  Out1 : Outport  InitialOutput=0
  wires:
  In1/1 -> Out1/1

== system shift_register_100/Enabled Subsystem46 ==
  In1 : Inport
  Enable : EnablePort
  Out1 : Outport  InitialOutput=0
  wires:
  In1/1 -> Out1/1

== system shift_register_100/Enabled Subsystem47 ==
  In1 : Inport
  Enable : EnablePort
  Out1 : Outport  InitialOutput=0
  wires:
  In1/1 -> Out1/1

== system shift_register_100/Enabled Subsystem48 ==
  In1 : Inport
  Enable : EnablePort
  Out1 : Outport  InitialOutput=0
  wires:
  In1/1 -> Out1/1

== system shift_register_100/Enabled Subsystem49 ==
  In1 : Inport
  Enable : EnablePort
  Out1 : Outport  InitialOutput=0
  wires:
  In1/1 -> Out1/1

== system shift_register_100/Enabled Subsystem5 ==
  In1 : Inport
  Enable : EnablePort
  Out1 : Outport  InitialOutput=0
  wires:
  In1/1 -> Out1/1

== system shift_register_100/Enabled Subsystem50 ==
  In1 : Inport
  Enable : EnablePort
  Out1 : Outport  InitialOutput=0
  wires:
  In1/1 -> Out1/1

== system shift_register_100/Enabled Subsystem51 ==
  In1 : Inport
  Enable : EnablePort
  Out1 : Outport  InitialOutput=0
  wires:
  In1/1 -> Out1/1

== system shift_register_100/Enabled Subsystem52 ==
  In1 : Inport
  Enable : EnablePort
  Out1 : Outport  InitialOutput=0
  wires:
  In1/1 -> Out1/1

== system shift_register_100/Enabled Subsystem53 ==
  In1 : Inport
  Enable : EnablePort
  Out1 : Outport  InitialOutput=0
  wires:
  In1/1 -> Out1/1

== system shift_register_100/Enabled Subsystem54 ==
  In1 : Inport
  Enable : EnablePort
  Out1 : Outport  InitialOutput=0
  wires:
  In1/1 -> Out1/1

== system shift_register_100/Enabled Subsystem55 ==
  In1 : Inport
  Enable : EnablePort
  Out1 : Outport  InitialOutput=0
  wires:
  In1/1 -> Out1/1

== system shift_register_100/Enabled Subsystem56 ==
  In1 : Inport
  Enable : EnablePort
  Out1 : Outport  InitialOutput=0
  wires:
  In1/1 -> Out1/1

== system shift_register_100/Enabled Subsystem57 ==
  In1 : Inport
  Enable : EnablePort
  Out1 : Outport  InitialOutput=0
  wires:
  In1/1 -> Out1/1

== system shift_register_100/Enabled Subsystem58 ==
  In1 : Inport
  Enable : EnablePort
  Out1 : Outport  InitialOutput=0
  wires:
  In1/1 -> Out1/1

== system shift_register_100/Enabled Subsystem59 ==
  In1 : Inport
  Enable : EnablePort
  Out1 : Outport  InitialOutput=0
  wires:
  In1/1 -> Out1/1

== system shift_register_100/Enabled Subsystem6 ==
  In1 : Inport
  Enable : EnablePort
  Out1 : Outport  InitialOutput=0
  wires:
  In1/1 -> Out1/1

== system shift_register_100/Enabled Subsystem60 ==
  In1 : Inport
  Enable : EnablePort
  Out1 : Outport  InitialOutput=0
  wires:
  In1/1 -> Out1/1

== system shift_register_100/Enabled Subsystem61 ==
  In1 : Inport
  Enable : EnablePort
  Out1 : Outport  InitialOutput=0
  wires:
  In1/1 -> Out1/1

== system shift_register_100/Enabled Subsystem62 ==
  In1 : Inport
  Enable : EnablePort
  Out1 : Outport  InitialOutput=0
  wires:
  In1/1 -> Out1/1

== system shift_register_100/Enabled Subsystem63 ==
  In1 : Inport
  Enable : EnablePort
  Out1 : Outport  InitialOutput=0
  wires:
  In1/1 -> Out1/1

== system shift_register_100/Enabled Subsystem64 ==
  In1 : Inport
  Enable : EnablePort
  Out1 : Outport  InitialOutput=0
  wires:
  In1/1 -> Out1/1

== system shift_register_100/Enabled Subsystem65 ==
  In1 : Inport
  Enable : EnablePort
  Out1 : Outport  InitialOutput=0
  wires:
  In1/1 -> Out1/1

== system shift_register_100/Enabled Subsystem66 ==
  In1 : Inport
  Enable : EnablePort
  Out1 : Outport  InitialOutput=0
  wires:
  In1/1 -> Out1/1

== system shift_register_100/Enabled Subsystem67 ==
  In1 : Inport
  Enable : EnablePort
  Out1 : Outport  InitialOutput=0
  wires:
  In1/1 -> Out1/1

== system shift_register_100/Enabled Subsystem68 ==
  In1 : Inport
  Enable : EnablePort
  Out1 : Outport  InitialOutput=0
  wires:
  In1/1 -> Out1/1

== system shift_register_100/Enabled Subsystem69 ==
  In1 : Inport
  Enable : EnablePort
  Out1 : Outport  InitialOutput=0
  wires:
  In1/1 -> Out1/1

== system shift_register_100/Enabled Subsystem7 ==
  In1 : Inport
  Enable : EnablePort
  Out1 : Outport  InitialOutput=0
  wires:
  In1/1 -> Out1/1

== system shift_register_100/Enabled Subsystem70 ==
  In1 : Inport
  Enable : EnablePort
  Out1 : Outport  InitialOutput=0
  wires:
  In1/1 -> Out1/1

== system shift_register_100/Enabled Subsystem71 ==
  In1 : Inport
  Enable : EnablePort
  Out1 : Outport  InitialOutput=0
  wires:
  In1/1 -> Out1/1

== system shift_register_100/Enabled Subsystem72 ==
  In1 : Inport
  Enable : EnablePort
  Out1 : Outport  InitialOutput=0
  wires:
  In1/1 -> Out1/1

== system shift_register_100/Enabled Subsystem73 ==
  In1 : Inport
  Enable : EnablePort
  Out1 : Outport  InitialOutput=0
  wires:
  In1/1 -> Out1/1

== system shift_register_100/Enabled Subsystem74 ==
  In1 : Inport
  Enable : EnablePort
  Out1 : Outport  InitialOutput=0
  wires:
  In1/1 -> Out1/1

== system shift_register_100/Enabled Subsystem75 ==
  In1 : Inport
  Enable : EnablePort
  Out1 : Outport  InitialOutput=0
  wires:
  In1/1 -> Out1/1

== system shift_register_100/Enabled Subsystem76 ==
  In1 : Inport
  Enable : EnablePort
  Out1 : Outport  InitialOutput=0
  wires:
  In1/1 -> Out1/1

== system shift_register_100/Enabled Subsystem77 ==
  In1 : Inport
  Enable : EnablePort
  Out1 : Outport  InitialOutput=0
  wires:
  In1/1 -> Out1/1

== system shift_register_100/Enabled Subsystem78 ==
  In1 : Inport
  Enable : EnablePort
  Out1 : Outport  InitialOutput=0
  wires:
  In1/1 -> Out1/1

== system shift_register_100/Enabled Subsystem79 ==
  In1 : Inport
  Enable : EnablePort
  Out1 : Outport  InitialOutput=0
  wires:
  In1/1 -> Out1/1

== system shift_register_100/Enabled Subsystem8 ==
  In1 : Inport
  Enable : EnablePort
  Out1 : Outport  InitialOutput=0
  wires:
  In1/1 -> Out1/1

== system shift_register_100/Enabled Subsystem80 ==
  In1 : Inport
  Enable : EnablePort
  Out1 : Outport  InitialOutput=0
  wires:
  In1/1 -> Out1/1

== system shift_register_100/Enabled Subsystem81 ==
  In1 : Inport
  Enable : EnablePort
  Out1 : Outport  InitialOutput=0
  wires:
  In1/1 -> Out1/1

== system shift_register_100/Enabled Subsystem82 ==
  In1 : Inport
  Enable : EnablePort
  Out1 : Outport  InitialOutput=0
  wires:
  In1/1 -> Out1/1

== system shift_register_100/Enabled Subsystem83 ==
  In1 : Inport
  Enable : EnablePort
  Out1 : Outport  InitialOutput=0
  wires:
  In1/1 -> Out1/1

== system shift_register_100/Enabled Subsystem84 ==
  In1 : Inport
  Enable : EnablePort
  Out1 : Outport  InitialOutput=0
  wires:
  In1/1 -> Out1/1

== system shift_register_100/Enabled Subsystem85 ==
  In1 : Inport
  Enable : EnablePort
  Out1 : Outport  InitialOutput=0
  wires:
  In1/1 -> Out1/1

== system shift_register_100/Enabled Subsystem86 ==
  In1 : Inport
  Enable : EnablePort
  Out1 : Outport  InitialOutput=0
  wires:
  In1/1 -> Out1/1

== system shift_register_100/Enabled Subsystem87 ==
  In1 : Inport
  Enable : EnablePort
  Out1 : Outport  InitialOutput=0
  wires:
  In1/1 -> Out1/1

== system shift_register_100/Enabled Subsystem88 ==
  In1 : Inport
  Enable : EnablePort
  Out1 : Outport  InitialOutput=0
  wires:
  In1/1 -> Out1/1

== system shift_register_100/Enabled Subsystem89 ==
  In1 : Inport
  Enable : EnablePort
  Out1 : Outport  InitialOutput=0
  wires:
  In1/1 -> Out1/1

== system shift_register_100/Enabled Subsystem9 ==
  In1 : Inport
  Enable : EnablePort
  Out1 : Outport  InitialOutput=0
  wires:
  In1/1 -> Out1/1

== system shift_register_100/Enabled Subsystem90 ==
  In1 : Inport
  Enable : EnablePort
  Out1 : Outport  InitialOutput=0
  wires:
  In1/1 -> Out1/1

== system shift_register_100/Enabled Subsystem91 ==
  In1 : Inport
  Enable : EnablePort
  Out1 : Outport  InitialOutput=0
  wires:
  In1/1 -> Out1/1

== system shift_register_100/Enabled Subsystem92 ==
  In1 : Inport
  Enable : EnablePort
  Out1 : Outport  InitialOutput=0
  wires:
  In1/1 -> Out1/1

== system shift_register_100/Enabled Subsystem93 ==
  In1 : Inport
  Enable : EnablePort
  Out1 : Outport  InitialOutput=0
  wires:
  In1/1 -> Out1/1

== system shift_register_100/Enabled Subsystem94 ==
  In1 : Inport
  Enable : EnablePort
  Out1 : Outport  InitialOutput=0
  wires:
  In1/1 -> Out1/1

== system shift_register_100/Enabled Subsystem95 ==
  In1 : Inport
  Enable : EnablePort
  Out1 : Outport  InitialOutput=0
  wires:
  In1/1 -> Out1/1

== system shift_register_100/Enabled Subsystem96 ==
  In1 : Inport
  Enable : EnablePort
  Out1 : Outport  InitialOutput=0
  wires:
  In1/1 -> Out1/1

== system shift_register_100/Enabled Subsystem97 ==
  In1 : Inport
  Enable : EnablePort
  Out1 : Outport  InitialOutput=0
  wires:
  In1/1 -> Out1/1

== system shift_register_100/Enabled Subsystem98 ==
  In1 : Inport
  Enable : EnablePort
  Out1 : Outport  InitialOutput=0
  wires:
  In1/1 -> Out1/1

== system shift_register_100/Enabled Subsystem99 ==
  In1 : Inport
  Enable : EnablePort
  Out1 : Outport  InitialOutput=0
  wires:
  In1/1 -> Out1/1
